simulink model "controller_model"  (R2018b)
settings: Solver=VariableStepAuto  StartTime=0.0  StopTime=Endtime  RelTol=1e-3
values from neighbouring files (symbols this model uses):
  alpha_A = (2^n - 1)/(V_A_max - V_A_min)    (= 204.6)    [controller_model_sim.m]
  alpha_i = 5/37.5    (= 0.133333333333)    [controller_model_sim.m]
  alpha_P = 100/(2^m - 1)    (= 0.392156862745)    [controller_model_sim.m]
  alpha_T = 1.5/1000    (= 0.0015)    [controller_model_sim.m]
  m = 8    [controller_model_sim.m]
  smp = 0.0001    [controller_model_sim.m]
  u_max = 100    [controller_model_sim.m]
  u_min = 0    [controller_model_sim.m]
  V_A_max = 5    [controller_model_sim.m]
  V_A_min = 0    [controller_model_sim.m]
  v_i_d = 1/12    (= 0.0833333333333)    [controller_model_sim.m]
  v_N_d = 1/12    (= 0.0833333333333)    [controller_model_sim.m]
libraries: simulink x2
settings Model: Creator=nharada  LastModifiedBy=nharada

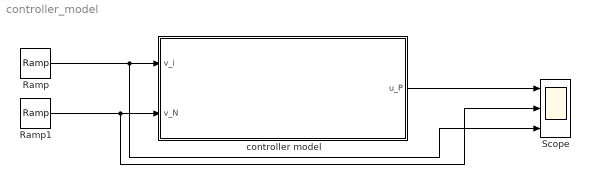
== system controller_model ==
  Ramp : simulink/Sources/Ramp  slope=v_i_d  start=0  InitialOutput=0
  Ramp1 : simulink/Sources/Ramp  slope=v_N_d  start=0  InitialOutput=0
  Scope : Scope  NumInputPorts=3
  controller model : Subsystem
  wires:
  Ramp1/1 -> Scope/2, controller model/2(v_N)
  Ramp/1 -> Scope/3, controller model/1(v_i)
  controller model/1(u_P) -> Scope/1

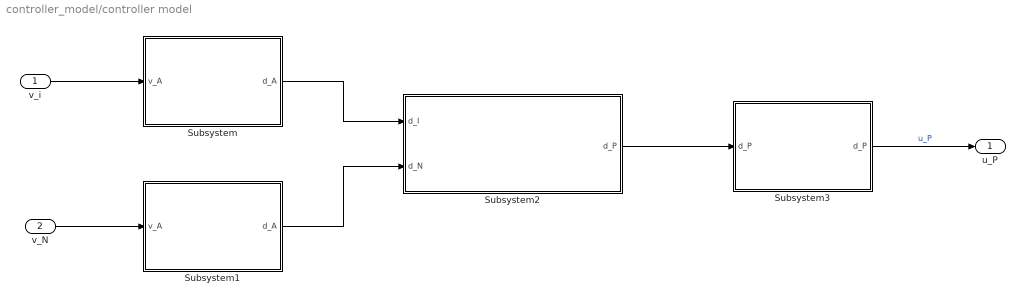
== system controller_model/controller model ==
  v_i : Inport
  v_N : Inport  Port=2
  Subsystem : Subsystem
  Subsystem1 : Subsystem
  Subsystem2 : Subsystem
  Subsystem3 : Subsystem
  u_P : Outport
  wires:
  Subsystem3/1(d_P) -> u_P/1  "u_P"
  Subsystem2/1(d_P) -> Subsystem3/1("d_P ")
  v_N/1 -> Subsystem1/1(v_A)
  Subsystem/1(d_A) -> Subsystem2/1(d_I)
  Subsystem1/1(d_A) -> Subsystem2/2(d_N)
  v_i/1 -> Subsystem/1(v_A)

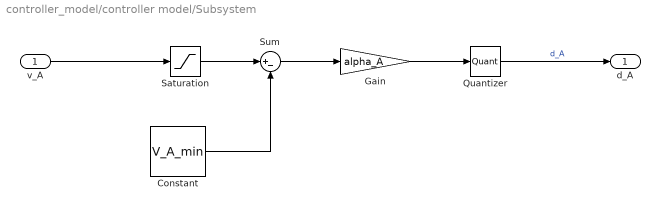
== system controller_model/controller model/Subsystem ==
  v_A : Inport
  Constant : Constant  Value=V_A_min  SampleTime=smp
  Gain : Gain  Gain=alpha_A
  Quantizer : Quantizer  QuantizationInterval=1
  Saturation : Saturate  UpperLimit=V_A_max  LowerLimit=V_A_min
  Sum : Sum  Inputs=|+-
  d_A : Outport
  wires:
  Saturation/1 -> Sum/1
  Constant/1 -> Sum/2
  Sum/1 -> Gain/1
  Gain/1 -> Quantizer/1
  v_A/1 -> Saturation/1
  Quantizer/1 -> d_A/1  "d_A"

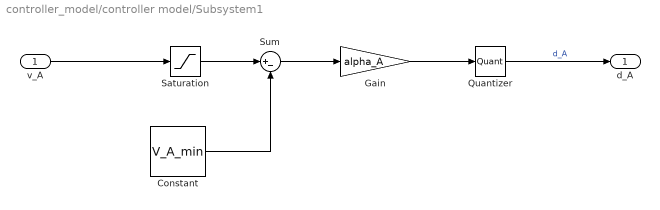
== system controller_model/controller model/Subsystem1 ==
  v_A : Inport
  Constant : Constant  Value=V_A_min  SampleTime=smp
  Gain : Gain  Gain=alpha_A
  Quantizer : Quantizer  QuantizationInterval=1
  Saturation : Saturate  UpperLimit=V_A_max  LowerLimit=V_A_min
  Sum : Sum  Inputs=|+-
  d_A : Outport
  wires:
  Saturation/1 -> Sum/1
  Constant/1 -> Sum/2
  Sum/1 -> Gain/1
  Gain/1 -> Quantizer/1
  v_A/1 -> Saturation/1
  Quantizer/1 -> d_A/1  "d_A"

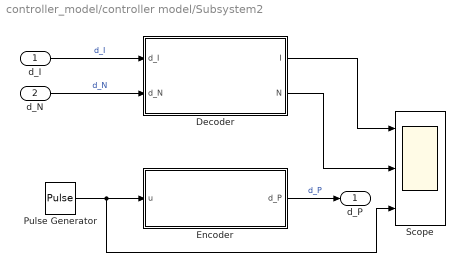
== system controller_model/controller model/Subsystem2 ==
  d_I : Inport
  d_N : Inport  Port=2
  Decoder : Subsystem
  Encoder : Subsystem
  Pulse Generator : DiscretePulseGenerator  PulseType=Time based  Amplitude=100  Period=30  PulseWidth=50
  Scope : Scope  NumInputPorts=3
  d_P : Outport
  wires:
  Pulse Generator/1 -> Scope/3, Encoder/1(u)
  Decoder/2(N) -> Scope/2
  d_N/1 -> Decoder/2(d_N)  "d_N"
  Decoder/1(I) -> Scope/1
  d_I/1 -> Decoder/1(d_I)  "d_I"
  Encoder/1(d_P) -> d_P/1  "d_P"

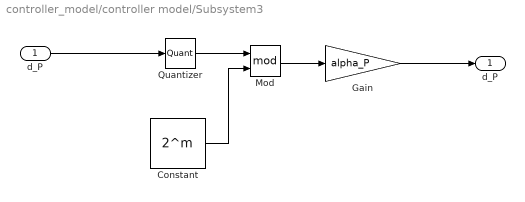
== system controller_model/controller model/Subsystem3 ==
  "d_P " : Inport
  Constant : Constant  Value=2^m  SampleTime=smp
  Gain : Gain  Gain=alpha_P
  Mod : Math  Operator=mod  SaturateOnIntegerOverflow=on
  Quantizer : Quantizer  QuantizationInterval=1
  d_P : Outport
  wires:
  Quantizer/1 -> Mod/1
  Constant/1 -> Mod/2
  Mod/1 -> Gain/1
  Gain/1 -> d_P/1
  "d_P "/1 -> Quantizer/1

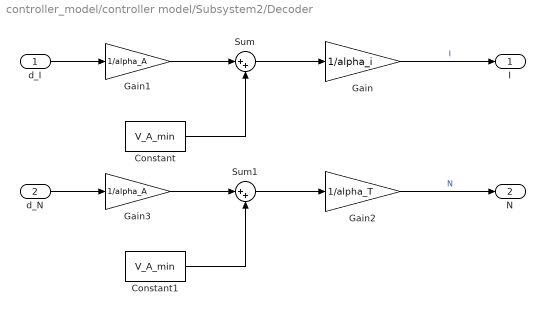
== system controller_model/controller model/Subsystem2/Decoder ==
  d_I : Inport
  d_N : Inport  Port=2
  Constant : Constant  Value=V_A_min  SampleTime=smp
  Constant1 : Constant  Value=V_A_min  SampleTime=smp
  Gain : Gain  Gain=1/alpha_i
  Gain1 : Gain  Gain=1/alpha_A
  Gain2 : Gain  Gain=1/alpha_T
  Gain3 : Gain  Gain=1/alpha_A
  Sum : Sum  Inputs=|++
  Sum1 : Sum  Inputs=|++
  I : Outport
  N : Outport  Port=2
  wires:
  Gain2/1 -> N/1  "N"
  Constant1/1 -> Sum1/2
  Gain/1 -> I/1  "I"
  Gain1/1 -> Sum/1
  d_N/1 -> Gain3/1
  Gain3/1 -> Sum1/1
  d_I/1 -> Gain1/1
  Constant/1 -> Sum/2
  Sum/1 -> Gain/1
  Sum1/1 -> Gain2/1

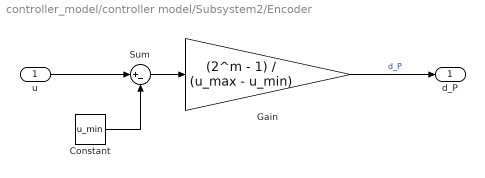
== system controller_model/controller model/Subsystem2/Encoder ==
  u : Inport
  Constant : Constant  Value=u_min  SampleTime=smp
  Gain : Gain  Gain=(2^m - 1) / (u_max - u_min)
  Sum : Sum  Inputs=|+-
  d_P : Outport
  wires:
  Sum/1 -> Gain/1
  Constant/1 -> Sum/2
  u/1 -> Sum/1
  Gain/1 -> d_P/1  "d_P"
